simulink model "hw1_q2"  (R2023b)
settings: Solver=VariableStepAuto  StartTime=0.0  StopTime=10.0  RelTol=1e-3
libraries: cstblocks x1, simulink x1
settings Model: Creator=ASUS  LastModifiedBy=mfb36

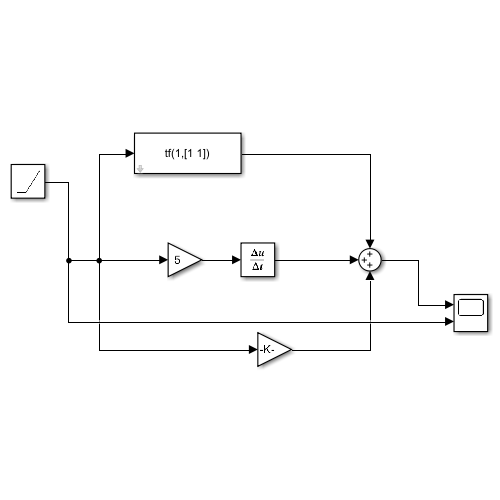
[thumbnail: Simulink's stored preview of the top-level diagram]
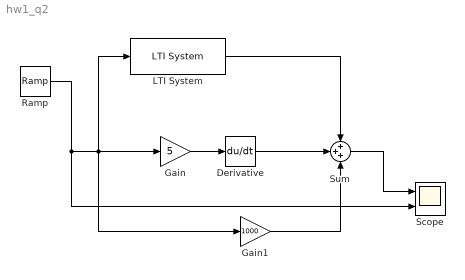
== system hw1_q2 ==
  Derivative : Derivative
  Gain : Gain  Gain=5
  Gain1 : Gain  Gain=1000
  LTI System : cstblocks/LTI System  sys=tf(1,[1 1])  IC=[]  PadeOrder=0
  Ramp : simulink/Sources/Ramp  slope=1  start=0  InitialOutput=0
  Scope : Scope  NumInputPorts=2
  Sum : Sum  Inputs=+++
  wires:
  Gain/1 -> Derivative/1
  Derivative/1 -> Sum/2
  Gain1/1 -> Sum/3
  Ramp/1 -> Scope/2, LTI System/1, Gain1/1, Gain/1
  Sum/1 -> Scope/1
  LTI System/1 -> Sum/1
